simulink model "stewart_kinematics"  (R2018a)
settings: Solver=VariableStepAuto  StartTime=0.0  StopTime=1  FixedStep=1e-6  RelTol=1e-3  EnableMultiTasking=on
values from neighbouring files (symbols this model uses):
  stewart = initializeParameters(stewart)    [params_micro_hexapod.m]    (also in params_nano_hexapod.m; stewart_parameters.m = struct())
  X = dmax.*cos(repmat(phi,length(theta),1)).*cos(repmat(theta,length(phi),1))'    [Position_max.m]    (also in getMaxPositions.m)
  Y = dmax.*cos(repmat(phi,length(theta),1)).*sin(repmat(theta,length(phi),1))'    [Position_max.m]    (also in getMaxPositions.m)
  Z = dmax.*sin(repmat(phi,length(theta),1))    [Position_max.m]    (also in getMaxPositions.m)
undefined symbols (not defined in the file or in its folder): sample
libraries: sm_lib x118, nesl_utility x66, simulink x1
(part 1 of 5)
settings Model: Creator=ThomasDehaeze  LastModifiedBy=DEHAEZE
settings DataIOCC: SaveOutput=off  SignalLogging=off  DSMLogging=off  SaveTime=off
settings OptimizationCC: LifeSpan=inf
settings DebuggingCC: AllowSymbolicDim=off  SFUnexpectedBacktrackingDiag=warning  SFNoUnconditionalDefaultTransitionDiag=warning  SFExecutionAtInitializationDiag=none
settings CodeAppCC: StateflowObjectComments=on
settings GRTTargetCC: TargetLangStandard=C89/C90 (ANSI)  GeneratePreprocessorConditionals=Disable all
settings ConfigComp: CovMetricSettings=dw  CovHtmlReporting=on  CovSaveCumulativeToWorkspaceVar=on  CovSaveSingleToWorkspaceVar=on  CovExternalEMLEnable=off  CovSFcnEnable=off
settings SimscapeCC: SimscapeNominalValues="[{\"value\":\"10\",\"unit\":\"V\"},{\"value\":\"1\",\"unit\":\"A\"},{\"value\":\"10\",\"unit\":\"N*m\"},{\"value\":\"10\",\"unit\":\"bar\"},{\"value\":\"100\",\"unit\":\"kJ/kg\"},{\"value\":\"1\",\"unit\":\"kW\"},{\"value\":\"300\",\"unit\":\"K\"},{\"value\":\"100\",\"unit\":\"cm^3/s\"},{\"value\":\"1\",\"unit\":\"kN\"},{\"value\":\"1\",\"unit\":\"g/cm^3\"},{\"value\":\"1\",\"unit\":\"l\"},{\"value\":\"1\",\"unit\":\"cm^2\"},{\"value\":\"60\",\"unit\":\"Hz\"}]"  SimscapeLogType=all  SimscapeLogDataHistory=10000
settings ConfigurationSet: Description=SimMechanics 2G

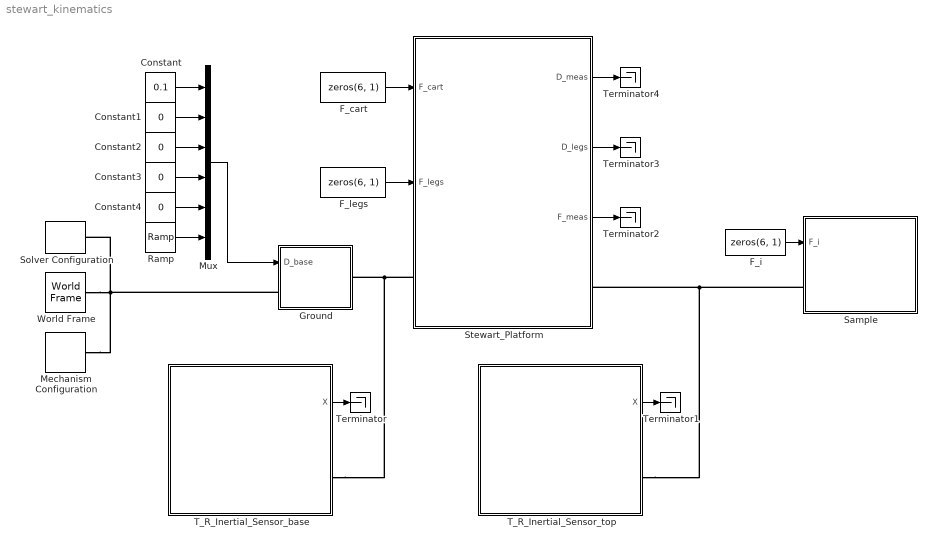
== system stewart_kinematics ==
  Constant : Constant  Value=0.1
  Constant{1..4} (4 alike) : Constant  Value=0
  F_cart : Constant  Value=zeros(6, 1)
  F_i : Constant  Value=zeros(6, 1)
  F_legs : Constant  Value=zeros(6, 1)
  Ground : Subsystem
  Mechanism Configuration : sm_lib/Utilities/Mechanism Configuration  UniformGravity=Constant  GravityVector=[0 0 0]  GravityUnits=m/s^2  LinearizationDelta=0.001
  Mux : Mux  Inputs=6
  Ramp : simulink/Sources/Ramp  slope=2*pi  start=0  InitialOutput=0
  Sample : Subsystem
      mask init:
      | load('./mat/sample.mat', 'sample');
  Solver Configuration : nesl_utility/Solver Configuration  PhysicalDomain=network_engine_domain  SubClassName=solver  LeftPortType=input  RightPortType=generic  Tones=[]  Harmonics=[]  SimulateNoise=off  Profile=off  UseLocalSampling=off  EnableSwitchedLinearOptims=on  FrequencyDomain=off  UseCCode=off  RelTol=0.001  AbsTol=1e-06  MinStep=1e-09  ToWorkspace=off  RevertToSquareIcSolve=off  NumHomotopyIterations=100  PhasorMode=off  PhasorModeNumHarmonics=1  DoDC=off  ResidualTolerance=1e-09  UseLocalSolver=off  LocalSolverChoice=NE_BACKWARD_EULER_ADVANCER  LocalSolverSampleTime=0.001  DoFixedCost=off  MaxNonlinIter=3  MaxModeIter=2  LinearAlgebra=Sparse  EquationFormulation=NE_TIME_EF  DelaysMemoryBudget=1024  AutomaticFiltering=on  FilteringTimeConstant=0.001
  Stewart_Platform : Subsystem
      mask init:
      | load('./mat/stewart.mat', 'stewart');
  T_R_Inertial_Sensor_base : Subsystem
  T_R_Inertial_Sensor_top : Subsystem
  Terminator{,1..4} (5 alike) : Terminator
  World Frame : sm_lib/Frames and Transforms/World Frame
  wires:
  F_cart/1 -> Stewart_Platform/1(F_cart)
  Stewart_Platform/1(D_meas) -> Terminator4/1
  Stewart_Platform/3(F_meas) -> Terminator2/1
  F_legs/1 -> Stewart_Platform/2(F_legs)
  Mux/1 -> Ground/1(D_base)
  F_i/1 -> Sample/1(F_i)
  T_R_Inertial_Sensor_base/1(X) -> Terminator/1
  T_R_Inertial_Sensor_top/1(X) -> Terminator1/1
  Stewart_Platform/2(D_legs) -> Terminator3/1
  Constant/1 -> Mux/1
  Constant1/1 -> Mux/2
  Constant2/1 -> Mux/3
  Constant3/1 -> Mux/4
  Constant4/1 -> Mux/5
  Ramp/1 -> Mux/6
  connections:
  Sample/LConn1 -- T_R_Inertial_Sensor_top/RConn1 -- Stewart_Platform/RConn1
  Mechanism Configuration/RConn1 -- Solver Configuration/RConn1 -- Ground/LConn1 -- World Frame/RConn1
  Stewart_Platform/LConn1 -- T_R_Inertial_Sensor_base/RConn1 -- Ground/RConn1

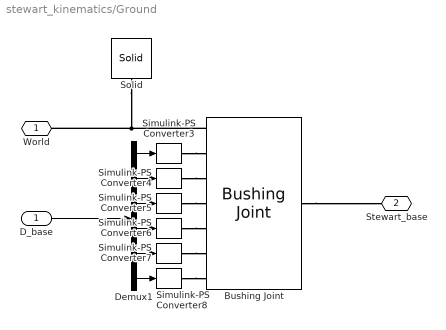
== system stewart_kinematics/Ground ==
  D_base : Inport
  Bushing Joint : sm_lib/Joints/Bushing Joint  SenseConstraintForce=off  SenseConstraintForceX=off  SenseConstraintForceY=off  SenseConstraintForceZ=off  SenseConstraintTorque=off  SenseConstraintTorqueX=off  SenseConstraintTorqueY=off  SenseConstraintTorqueZ=off  SenseTotalForce=off  SenseTotalForceX=off  SenseTotalForceY=off  SenseTotalForceZ=off  SenseTotalTorque=off  SenseTotalTorqueX=off  SenseTotalTorqueY=off  SenseTotalTorqueZ=off  CompositeWrenchDir=FollowerOnBase  CompositeWrenchFrame=BaseFrame  PxEquilibriumPosition=0  PxEquilibriumPositionUnits=m  PxSpringStiffness=0  PxSpringStiffnessUnits=N/m  PxDampingCoefficient=0  PxDampingCoefficientUnits=N/(m/s)  PxTorqueActuationMode=ComputedTorque  PxMotionActuationMode=InputMotion  PxSensePosition=off  PxSenseVelocity=off  PxSenseAcceleration=off  PxSenseTorqueForce=off  PxPositionTargetSpecify=off  PxPositionTargetPriority=High  PxPositionTargetValue=0  PxPositionTargetValueUnits=m  PxVelocityTargetSpecify=off  PxVelocityTargetPriority=High  PxVelocityTargetValue=0  PxVelocityTargetValueUnits=m/s  PyEquilibriumPosition=0  PyEquilibriumPositionUnits=m  PySpringStiffness=0  PySpringStiffnessUnits=N/m  PyDampingCoefficient=0  PyDampingCoefficientUnits=N/(m/s)  PyTorqueActuationMode=ComputedTorque  PyMotionActuationMode=InputMotion  PySensePosition=off  PySenseVelocity=off  PySenseAcceleration=off  PySenseTorqueForce=off  PyPositionTargetSpecify=off  PyPositionTargetPriority=High  PyPositionTargetValue=0  PyPositionTargetValueUnits=m  PyVelocityTargetSpecify=off  PyVelocityTargetPriority=High  PyVelocityTargetValue=0  PyVelocityTargetValueUnits=m/s  PzEquilibriumPosition=0  PzEquilibriumPositionUnits=m  PzSpringStiffness=0  PzSpringStiffnessUnits=N/m  PzDampingCoefficient=0  PzDampingCoefficientUnits=N/(m/s)  PzTorqueActuationMode=ComputedTorque  PzMotionActuationMode=InputMotion  PzSensePosition=off  PzSenseVelocity=off  PzSenseAcceleration=off  PzSenseTorqueForce=off  PzPositionTargetSpecify=off  PzPositionTargetPriority=High  PzPositionTargetValue=0  PzPositionTargetValueUnits=m  PzVelocityTargetSpecify=off  PzVelocityTargetPriority=High  PzVelocityTargetValue=0  PzVelocityTargetValueUnits=m/s  RxEquilibriumPosition=0  RxEquilibriumPositionUnits=deg  RxSpringStiffness=0  RxSpringStiffnessUnits=N*m/deg  RxDampingCoefficient=0  RxDampingCoefficientUnits=N*m/(deg/s)  RxTorqueActuationMode=ComputedTorque  RxMotionActuationMode=InputMotion  RxSensePosition=off  RxSenseVelocity=off  RxSenseAcceleration=off  RxSenseTorqueForce=off  RxPositionTargetSpecify=off  RxPositionTargetPriority=High  RxPositionTargetValue=0  RxPositionTargetValueUnits=deg  RxVelocityTargetSpecify=off  RxVelocityTargetPriority=High  RxVelocityTargetValue=0  RxVelocityTargetValueUnits=deg/s  RyEquilibriumPosition=0  RyEquilibriumPositionUnits=deg  RySpringStiffness=0  RySpringStiffnessUnits=N*m/deg  RyDampingCoefficient=0  RyDampingCoefficientUnits=N*m/(deg/s)  RyTorqueActuationMode=ComputedTorque  RyMotionActuationMode=InputMotion  RySensePosition=off  RySenseVelocity=off  RySenseAcceleration=off  RySenseTorqueForce=off  RyPositionTargetSpecify=off  RyPositionTargetPriority=High  RyPositionTargetValue=0  RyPositionTargetValueUnits=deg  RyVelocityTargetSpecify=off  RyVelocityTargetPriority=High  RyVelocityTargetValue=0  RyVelocityTargetValueUnits=deg/s  RzEquilibriumPosition=0  RzEquilibriumPositionUnits=deg  RzSpringStiffness=0  RzSpringStiffnessUnits=N*m/deg  RzDampingCoefficient=0  RzDampingCoefficientUnits=N*m/(deg/s)  RzTorqueActuationMode=ComputedTorque  RzMotionActuationMode=InputMotion  RzSensePosition=off  RzSenseVelocity=off  RzSenseAcceleration=off  RzSenseTorqueForce=off  RzPositionTargetSpecify=off  RzPositionTargetPriority=High  RzPositionTargetValue=0  RzPositionTargetValueUnits=deg  RzVelocityTargetSpecify=off  RzVelocityTargetPriority=High  RzVelocityTargetValue=0  RzVelocityTargetValueUnits=deg/s
      settings: SourceProductName=Simscape Multibody
  Demux1 : Demux  Outputs=6
  Simulink-PS Converter{3..8} (6 alike) : nesl_utility/Simulink-PS Converter  PhysicalDomain=network_engine_domain  SubClassName=ps_input  LeftPortType=input  RightPortType=output  PseudoPeriodic=off  Frequencies=[]  NoiseDistribution=none  NoiseParameters=[]  Unit=1  AffineConversion=off  FilteringAndDerivatives=filter  SimscapeFilterOrder=2  InputFilterTimeConstant=0.0001  UdotUserProvided=0
  Solid : sm_lib/Body Elements/Solid  InertiaType=CalculateFromGeometry  Mass=1  MassUnits=kg  CenterOfMass=[0 0 0]  CenterOfMassUnits=m  MomentsOfInertia=[1 1 1]  MomentsOfInertiaUnits=kg*m^2  ProductsOfInertia=[0 0 0]  ProductsOfInertiaUnits=kg*m^2  DensityBased=on  Density=1000  DensityUnits=kg/m^3  DoExposeReferenceFrame=off  SerializedFrames=<Frames><Frame><Id>Frame1</Id><Value><Name>F1</Name><Origin><Source>GeometricFeature</Source><FeatureName>top surface</FeatureName></Origin><PrimaryAxis><DefinedDirection>+Z</DefinedDirection><Source>ReferenceFrame</Source><SourceDirection>+Z</SourceDirection><FeatureName></FeatureName></PrimaryAxis><SecondaryAxis><DefinedDirection>+X</DefinedDirection><Source>ReferenceFrame</Source><SourceDirection>+X</SourceDirection><FeatureName></FeatureName></SecondaryAxis></Value></Frame></Frames>  GraphicType=FromGeometry  MarkerShape=Sphere  MarkerSize=10  GraphicVisPropType=SimpleVisualProperties  GraphicDiffuseColor=[0.5 0.5 0.5]  GraphicSpecularColor=[0.5 0.5 0.5 1.0]  GraphicAmbientColor=[0.15 0.15 0.15 1.0]  GraphicEmissiveColor=[0.0 0.0 0.0 1.0]  GraphicShininess=75  GraphicOpacity=1.0  GeometryShape=Cylinder  RectangleSize=[1 1]  RectangleSizeUnits=m  BrickDimensions=[1 1 0.1]  BrickDimensionUnits=m  CylinderRadius=0.5  CylinderRadiusUnits=m  CylinderLength=0.1  CylinderLengthUnits=m  SphereRadius=1  SphereRadiusUnits=m  EllipsoidRadii=[1 1 1]  EllipsoidRadiiUnits=m  ExtrusionCrossSection=[1 1; -1 1; -1 -1; 1 -1]  ExtrusionCrossSectionUnits=m  ExtrusionLength=1  ExtrusionLengthUnits=m  PolygonNumSides=3  PolygonOuterRadius=1  PolygonOuterRadiusUnits=m  ExtGeomFileType=STEP  ExtGeomFileUnits=m  RevolutionCrossSection=[1 1; 1 -1; 2 -1; 2 1]  RevolutionCrossSectionUnits=m  RevolutionExtent=Full  RevolutionAngle=180  RevolutionAngleUnits=deg
  World : PMIOPort  Side=Left
  Stewart_base : PMIOPort  Port=2  Side=Right
  wires:
  Demux1/1 -> Simulink-PS Converter3/1
  Demux1/2 -> Simulink-PS Converter4/1
  Demux1/3 -> Simulink-PS Converter5/1
  Demux1/4 -> Simulink-PS Converter6/1
  Demux1/5 -> Simulink-PS Converter7/1
  Demux1/6 -> Simulink-PS Converter8/1
  D_base/1 -> Demux1/1
  connections:
  Bushing Joint/RConn1 -- Stewart_base/RConn1
  Solid/LConn1 -- World/RConn1 -- Bushing Joint/LConn1
  Simulink-PS Converter3/RConn1 -- Bushing Joint/LConn2
  Simulink-PS Converter4/RConn1 -- Bushing Joint/LConn3
  Simulink-PS Converter5/RConn1 -- Bushing Joint/LConn4
  Simulink-PS Converter8/RConn1 -- Bushing Joint/LConn7
  Simulink-PS Converter7/RConn1 -- Bushing Joint/LConn6
  Simulink-PS Converter6/RConn1 -- Bushing Joint/LConn5

== system stewart_kinematics/Sample ==
  note: Sample
  note: X-Offset for the Sample
  F_i : Inport
  Eternal_Force_and_Torque : Subsystem
  Rigid Transform : sm_lib/Frames and Transforms/Rigid Transform  TranslationMethod=StandardAxis  TranslationStandardOffset=sample.offset  TranslationLengthUnit=mm  TranslationStandardAxis=+X  TranslationCartesianOffset=[0 0 0]  TranslationROffset=0  TranslationROffsetUnits=m  TranslationZOffset=0  TranslationZOffsetUnits=m  TranslationThetaOffset=0  TranslationThetaOffsetUnits=deg  RotationMethod=None  RotationAngleUnits=deg  RotationStandardAxis=+Z  RotationAngle=0.0  RotationArbitraryAxis=[0 0 1]  FollAlignAxisA=+X  BaseAlignAxisA=+Y  FollAlignAxisB=+Y  BaseAlignAxisB=+Z  RotationSequenceAxes=FollowerAxes  RotationSequence=XYX  RotationSequenceAngles=[0 0 0]  RotationSequenceAnglesUnits=deg  RotationMatrix=[1 0 0; 0 1 0; 0 0 1]
  Solid1 : sm_lib/Body Elements/Solid  InertiaType=CalculateFromGeometry  Mass=sample.mass  MassUnits=kg  CenterOfMass=[0 0 0]  CenterOfMassUnits=m  MomentsOfInertia=[1 1 1]  MomentsOfInertiaUnits=kg*m^2  ProductsOfInertia=[1 1 1]  ProductsOfInertiaUnits=kg*m^2  DensityBased=off  Density=1000  DensityUnits=kg/m^3  DoExposeReferenceFrame=on  SerializedFrames=<Frames><Frame><Id>Frame1</Id><Value><Name>F1</Name><Origin><Source>GeometricFeature</Source><FeatureName>bottom surface</FeatureName></Origin><PrimaryAxis><DefinedDirection>+Z</DefinedDirection><Source>ReferenceFrame</Source><SourceDirection>+Z</SourceDirection><FeatureName></FeatureName></PrimaryAxis><SecondaryAxis><DefinedDirection>+X</DefinedDirection><Source>ReferenceFrame</Source><SourceDirection>+X</SourceDirection><FeatureName></FeatureName></SecondaryAxis></Value></Frame></Frames>  GraphicType=FromGeometry  MarkerShape=Sphere  MarkerSize=10  GraphicVisPropType=SimpleVisualProperties  GraphicDiffuseColor=sample.color  GraphicSpecularColor=[0.5 0.5 0.5 1.0]  GraphicAmbientColor=[0.15 0.15 0.15 1.0]  GraphicEmissiveColor=[0.0 0.0 0.0 1.0]  GraphicShininess=75  GraphicOpacity=1.0  GeometryShape=Cylinder  RectangleSize=[1 1]  RectangleSizeUnits=m  BrickDimensions=[1 1 1]  BrickDimensionUnits=m  CylinderRadius=sample.radius  CylinderRadiusUnits=mm  CylinderLength=sample.height  CylinderLengthUnits=mm  SphereRadius=1  SphereRadiusUnits=m  EllipsoidRadii=[1 1 1]  EllipsoidRadiiUnits=m  ExtrusionCrossSection=[1 1; -1 1; -1 -1; 1 -1]  ExtrusionCrossSectionUnits=m  ExtrusionLength=1  ExtrusionLengthUnits=m  PolygonNumSides=3  PolygonOuterRadius=1  PolygonOuterRadiusUnits=m  ExtGeomFileType=STEP  ExtGeomFileUnits=m  RevolutionCrossSection=[1 1; 1 -1; 2 -1; 2 1]  RevolutionCrossSectionUnits=m  RevolutionExtent=Full  RevolutionAngle=180  RevolutionAngleUnits=deg
  Sample_bot : PMIOPort  Side=Left
  wires:
  F_i/1 -> Eternal_Force_and_Torque/1(F_ext)
  connections:
  Solid1/LConn1 -- Rigid Transform/RConn1
  Sample_bot/RConn1 -- Rigid Transform/LConn1
  Eternal_Force_and_Torque/RConn1 -- Solid1/RConn1

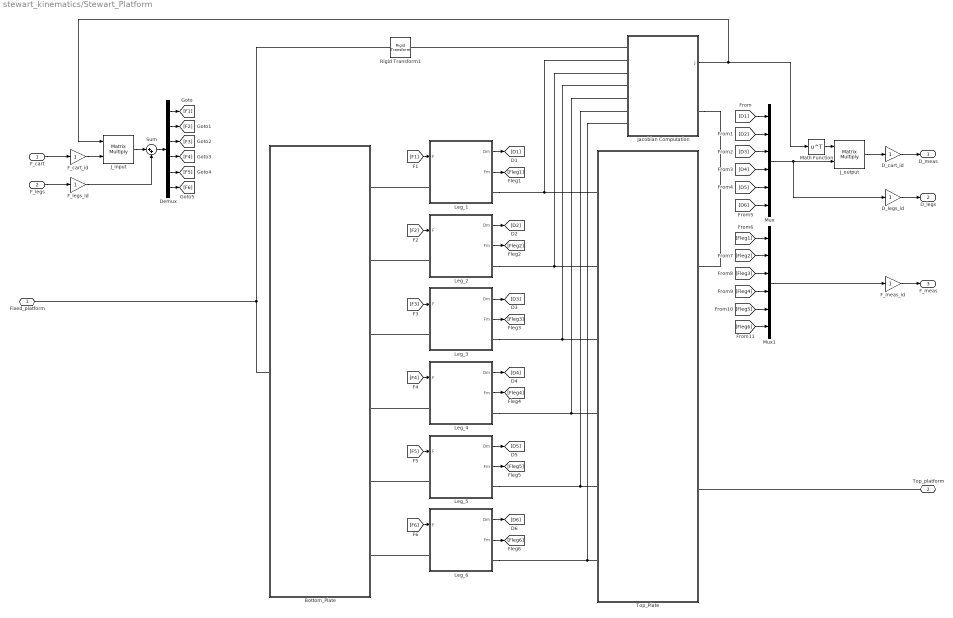
== system stewart_kinematics/Stewart_Platform ==
  F_cart : Inport
  F_legs : Inport  Port=2
  Bottom_Plate : Subsystem
  D_cart_id : Gain
  D_legs_id : Gain
  Demux : Demux  Outputs=6
  F_cart_id : Gain
  F_legs_id : Gain
  F_meas_id : Gain
  J_input : Product  Multiplication=Matrix(*)
  J_output : Product  Multiplication=Matrix(*)
  Jacobian Computation : Subsystem
  Leg_1 : Subsystem
  Leg_2 : Subsystem
  Leg_3 : Subsystem
  Leg_4 : Subsystem
  Leg_5 : Subsystem
  Leg_6 : Subsystem
  Math Function : Math  Operator=transpose  SaturateOnIntegerOverflow=on
  Mux : Mux  Inputs=6
  Mux1 : Mux  Inputs=6
  Rigid Transform1 : sm_lib/Frames and Transforms/Rigid Transform  TranslationMethod=StandardAxis  TranslationStandardOffset=stewart.jacobian+stewart.h  TranslationLengthUnit=mm  TranslationStandardAxis=+Z  TranslationCartesianOffset=[0 0 0]  TranslationROffset=0  TranslationROffsetUnits=m  TranslationZOffset=0  TranslationZOffsetUnits=m  TranslationThetaOffset=0  TranslationThetaOffsetUnits=deg  RotationMethod=None  RotationAngleUnits=deg  RotationStandardAxis=+Z  RotationAngle=0.0  RotationArbitraryAxis=[0 0 1]  FollAlignAxisA=+X  BaseAlignAxisA=+Y  FollAlignAxisB=+Y  BaseAlignAxisB=+Z  RotationSequenceAxes=FollowerAxes  RotationSequence=XYX  RotationSequenceAngles=[0 0 0]  RotationSequenceAnglesUnits=deg  RotationMatrix=[1 0 0; 0 1 0; 0 0 1]
  Sum : Sum  Inputs=|++
  Top_Plate : Subsystem
  Fixed_platform : PMIOPort  Side=Left
  Top_platform : PMIOPort  Port=2  Side=Right
  D_meas : Outport
  D_legs : Outport  Port=2
  F_meas : Outport  Port=3
  wires:
  Demux/1 -> [F1]
  [F3] -> Leg_3/1(F)
  [F5] -> Leg_5/1(F)
  Demux/4 -> [F4]
  Demux/2 -> [F2]
  Leg_5/1(Dm) -> [D5]
  Leg_3/1(Dm) -> [D3]
  Demux/5 -> [F5]
  Demux/6 -> [F6]
  [F6] -> Leg_6/1(F)
  [F4] -> Leg_4/1(F)
  Demux/3 -> [F3]
  Leg_4/1(Dm) -> [D4]
  Leg_2/1(Dm) -> [D2]
  [F2] -> Leg_2/1(F)
  Leg_6/1(Dm) -> [D6]
  F_cart/1 -> F_cart_id/1
  Jacobian Computation/1(J) -> J_input/1, Math Function/1
  J_input/1 -> Sum/1
  [D3] -> Mux/3
  J_output/1 -> D_cart_id/1
  [D5] -> Mux/5
  Mux/1 -> D_legs_id/1, J_output/2
  Math Function/1 -> J_output/1
  [D6] -> Mux/6
  [D1] -> Mux/1
  [D4] -> Mux/4
  [D2] -> Mux/2
  [F1] -> Leg_1/1(F)
  Leg_1/1(Dm) -> [D1]
  Sum/1 -> Demux/1
  F_legs/1 -> F_legs_id/1
  D_legs_id/1 -> D_legs/1
  D_cart_id/1 -> D_meas/1
  F_legs_id/1 -> Sum/2
  F_cart_id/1 -> J_input/2
  Leg_2/2(Fm) -> [Fleg2]
  Leg_3/2(Fm) -> [Fleg3]
  Leg_4/2(Fm) -> [Fleg4]
  Leg_5/2(Fm) -> [Fleg5]
  Leg_6/2(Fm) -> [Fleg6]
  Leg_1/2(Fm) -> [Fleg1]
  [Fleg1] -> Mux1/1
  [Fleg2] -> Mux1/2
  [Fleg3] -> Mux1/3
  [Fleg4] -> Mux1/4
  [Fleg5] -> Mux1/5
  [Fleg6] -> Mux1/6
  F_meas_id/1 -> F_meas/1
  Mux1/1 -> F_meas_id/1
  connections:
  Jacobian Computation/LConn3 -- Leg_2/RConn1 -- Top_Plate/LConn2
  Leg_4/LConn1 -- Bottom_Plate/RConn4
  Jacobian Computation/LConn5 -- Leg_4/RConn1 -- Top_Plate/LConn4
  Top_Plate/LConn1 -- Leg_1/RConn1 -- Jacobian Computation/LConn2
  Leg_3/LConn1 -- Bottom_Plate/RConn3
  Jacobian Computation/LConn4 -- Top_Plate/LConn3 -- Leg_3/RConn1
  Jacobian Computation/LConn6 -- Leg_5/RConn1 -- Top_Plate/LConn5
  Leg_2/LConn1 -- Bottom_Plate/RConn2
  Leg_5/LConn1 -- Bottom_Plate/RConn5
  Leg_1/LConn1 -- Bottom_Plate/RConn1
  Jacobian Computation/LConn7 -- Leg_6/RConn1 -- Top_Plate/LConn6
  Leg_6/LConn1 -- Bottom_Plate/RConn6
  Top_platform/RConn1 -- Top_Plate/RConn2
  Jacobian Computation/RConn1 -- Top_Plate/RConn1
  Rigid Transform1/LConn1 -- Bottom_Plate/LConn1 -- Fixed_platform/RConn1
  Jacobian Computation/LConn1 -- Rigid Transform1/RConn1

== system stewart_kinematics/T_R_Inertial_Sensor_base ==
  Model : ModelReference  ModelNameDialog=QuaternionToAngles.slx  SimulationMode=Normal  ModelReferenceVersion=1.10
  Mux : Mux  Inputs=6
  PS-Simulink Converter{1,3..5} (4 alike) : nesl_utility/PS-Simulink Converter  PhysicalDomain=network_engine_domain  SubClassName=ps_output  LeftPortType=input  RightPortType=output  PseudoPeriodic=off  Frequencies=[]  Unit=1  AffineConversion=off
  Transform Sensor : sm_lib/Frames and Transforms/Transform Sensor  MeasurementFrame=Base  SenseAngle=off  SenseAxis=off  SenseAngle1=off  SenseAngle2=off  SenseAngle3=off  SenseQ=on  SenseR=off  SenseOmegaX=off  SenseOmegaY=off  SenseOmegaZ=off  SenseOmega1=off  SenseOmega2=off  SenseOmega3=off  SenseQDot=off  SenseRDot=off  SenseAlphaX=off  SenseAlphaY=off  SenseAlphaZ=off  SenseAlpha1=off  SenseAlpha2=off  SenseAlpha3=off  SenseQDDot=off  SenseRDDot=off  SenseX=on  SenseY=on  SenseZ=on  SenseRad=off  SenseAzim=off  SenseDist=off  SenseInc=off  SenseXDot=off  SenseYDot=off  SenseZDot=off  SenseRadDot=off  SenseAzimDot=off  SenseDistDot=off  SenseIncDot=off  SenseXDDot=off  SenseYDDot=off  SenseZDDot=off  SenseRadDDot=off  SenseAzimDDot=off  SenseDistDDot=off  SenseIncDDot=off
  World Frame1 : sm_lib/Frames and Transforms/World Frame
  F : PMIOPort  Side=Right
  X : Outport
  wires:
  PS-Simulink Converter4/1 -> Mux/2  "y"
  PS-Simulink Converter3/1 -> Mux/1  "x"
  PS-Simulink Converter1/1 -> Model/1
  Model/1 -> Mux/4
  Model/2 -> Mux/5
  Model/3 -> Mux/6
  PS-Simulink Converter5/1 -> Mux/3  "z"
  Mux/1 -> X/1
  connections:
  World Frame1/RConn1 -- Transform Sensor/LConn1
  Transform Sensor/RConn1 -- F/RConn1
  Transform Sensor/RConn5 -- PS-Simulink Converter5/LConn1
  Transform Sensor/RConn3 -- PS-Simulink Converter3/LConn1
  Transform Sensor/RConn4 -- PS-Simulink Converter4/LConn1
  PS-Simulink Converter1/LConn1 -- Transform Sensor/RConn2

== system stewart_kinematics/T_R_Inertial_Sensor_top ==
  Model : ModelReference  ModelNameDialog=QuaternionToAngles.slx  SimulationMode=Normal  ModelReferenceVersion=1.10
  Mux : Mux  Inputs=6
  PS-Simulink Converter{1,3..5} (4 alike) : nesl_utility/PS-Simulink Converter  PhysicalDomain=network_engine_domain  SubClassName=ps_output  LeftPortType=input  RightPortType=output  PseudoPeriodic=off  Frequencies=[]  Unit=1  AffineConversion=off
  Transform Sensor : sm_lib/Frames and Transforms/Transform Sensor  MeasurementFrame=Base  SenseAngle=off  SenseAxis=off  SenseAngle1=off  SenseAngle2=off  SenseAngle3=off  SenseQ=on  SenseR=off  SenseOmegaX=off  SenseOmegaY=off  SenseOmegaZ=off  SenseOmega1=off  SenseOmega2=off  SenseOmega3=off  SenseQDot=off  SenseRDot=off  SenseAlphaX=off  SenseAlphaY=off  SenseAlphaZ=off  SenseAlpha1=off  SenseAlpha2=off  SenseAlpha3=off  SenseQDDot=off  SenseRDDot=off  SenseX=on  SenseY=on  SenseZ=on  SenseRad=off  SenseAzim=off  SenseDist=off  SenseInc=off  SenseXDot=off  SenseYDot=off  SenseZDot=off  SenseRadDot=off  SenseAzimDot=off  SenseDistDot=off  SenseIncDot=off  SenseXDDot=off  SenseYDDot=off  SenseZDDot=off  SenseRadDDot=off  SenseAzimDDot=off  SenseDistDDot=off  SenseIncDDot=off
  World Frame1 : sm_lib/Frames and Transforms/World Frame
  F : PMIOPort  Side=Right
  X : Outport
  wires:
  Mux/1 -> X/1
  PS-Simulink Converter5/1 -> Mux/3  "z"
  Model/3 -> Mux/6
  Model/2 -> Mux/5
  Model/1 -> Mux/4
  PS-Simulink Converter1/1 -> Model/1
  PS-Simulink Converter3/1 -> Mux/1  "x"
  PS-Simulink Converter4/1 -> Mux/2  "y"
  connections:
  PS-Simulink Converter1/LConn1 -- Transform Sensor/RConn2
  Transform Sensor/RConn4 -- PS-Simulink Converter4/LConn1
  Transform Sensor/RConn3 -- PS-Simulink Converter3/LConn1
  Transform Sensor/RConn5 -- PS-Simulink Converter5/LConn1
  Transform Sensor/RConn1 -- F/RConn1
  World Frame1/RConn1 -- Transform Sensor/LConn1

== system stewart_kinematics/Sample/Eternal_Force_and_Torque ==
  F_ext : Inport  PortDimensions=6
  Demux1 : Demux  Outputs=6
  External Force and Torque1 : sm_lib/Forces and Torques/External Force and Torque  ForceResolutionFrame=World  EnableForceX=on  EnableForceY=on  EnableForceZ=on  EnableForce=off  TorqueResolutionFrame=AttachedFrame  EnableTorqueX=on  EnableTorqueY=on  EnableTorqueZ=on  EnableTorque=off
  Simulink-PS Converter{1..6} (6 alike) : nesl_utility/Simulink-PS Converter  PhysicalDomain=network_engine_domain  SubClassName=ps_input  LeftPortType=input  RightPortType=output  PseudoPeriodic=off  Frequencies=[]  NoiseDistribution=none  NoiseParameters=[]  Unit=1  AffineConversion=off  FilteringAndDerivatives=provide  SimscapeFilterOrder=1  InputFilterTimeConstant=0.001  UdotUserProvided=0
  F : PMIOPort  Side=Right
  wires:
  Demux1/2 -> Simulink-PS Converter4/1
  Demux1/1 -> Simulink-PS Converter3/1
  Demux1/3 -> Simulink-PS Converter5/1
  F_ext/1 -> Demux1/1
  Demux1/6 -> Simulink-PS Converter6/1
  Demux1/4 -> Simulink-PS Converter1/1
  Demux1/5 -> Simulink-PS Converter2/1
  connections:
  F/RConn1 -- External Force and Torque1/RConn1
  Simulink-PS Converter4/RConn1 -- External Force and Torque1/LConn2
  Simulink-PS Converter5/RConn1 -- External Force and Torque1/LConn3
  Simulink-PS Converter3/RConn1 -- External Force and Torque1/LConn1
  Simulink-PS Converter1/RConn1 -- External Force and Torque1/LConn4
  Simulink-PS Converter2/RConn1 -- External Force and Torque1/LConn5
  Simulink-PS Converter6/RConn1 -- External Force and Torque1/LConn6

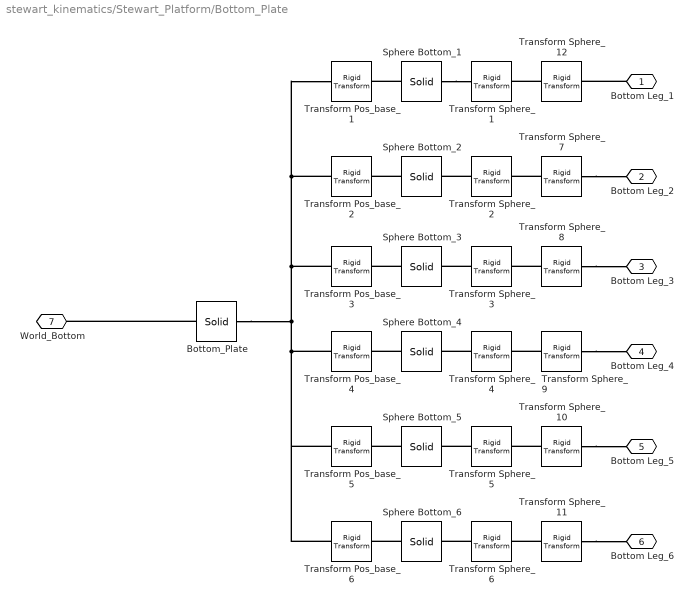
== system stewart_kinematics/Stewart_Platform/Bottom_Plate ==
  Bottom_Plate : sm_lib/Body Elements/Solid  InertiaType=CalculateFromGeometry  Mass=1  MassUnits=kg  CenterOfMass=[0 0 0]  CenterOfMassUnits=m  MomentsOfInertia=[1 1 1]  MomentsOfInertiaUnits=kg*m^2  ProductsOfInertia=[1 1 1]  ProductsOfInertiaUnits=kg*m^2  DensityBased=on  Density=stewart.BP.density  DensityUnits=kg/m^3  DoExposeReferenceFrame=on  SerializedFrames=<Frames><Frame><Id>Frame1</Id><Value><Name>T</Name><Origin><Source>GeometricFeature</Source><FeatureName>side surface 4</FeatureName></Origin><PrimaryAxis><DefinedDirection>+Z</DefinedDirection><Source>ReferenceFrame</Source><SourceDirection>+Z</SourceDirection><FeatureName></FeatureName></PrimaryAxis><SecondaryAxis><DefinedDirection>+X</DefinedDirection><Source>ReferenceFrame</Source><SourceDirection>+X</SourceDirection><FeatureName></FeatureName></SecondaryAxis></Value></Frame></Frames>  GraphicType=FromGeometry  MarkerShape=Sphere  MarkerSize=10  GraphicVisPropType=SimpleVisualProperties  GraphicDiffuseColor=stewart.BP.color  GraphicSpecularColor=[0.5 0.5 0.5 1.0]  GraphicAmbientColor=[0.15 0.15 0.15 1.0]  GraphicEmissiveColor=[0.0 0.0 0.0 1.0]  GraphicShininess=75  GraphicOpacity=1.0  GeometryShape=GeneralSolidOfRevolution  RectangleSize=[1 1]  RectangleSizeUnits=m  BrickDimensions=[1 1 1]  BrickDimensionUnits=m  CylinderRadius=1  CylinderRadiusUnits=m  CylinderLength=1  CylinderLengthUnits=m  SphereRadius=1  SphereRadiusUnits=m  EllipsoidRadii=[1 1 1]  EllipsoidRadiiUnits=m  ExtrusionCrossSection=[1 1; -1 1; -1 -1; 1 -1]  ExtrusionCrossSectionUnits=m  ExtrusionLength=1  ExtrusionLengthUnits=m  PolygonNumSides=3  PolygonOuterRadius=1  PolygonOuterRadiusUnits=m  ExtGeomFileType=STEP  ExtGeomFileUnits=m  RevolutionCrossSection=stewart.BP.shape  RevolutionCrossSectionUnits=mm  RevolutionExtent=Full  RevolutionAngle=180  RevolutionAngleUnits=deg
  Sphere Bottom_{1..6} (6 alike) : sm_lib/Body Elements/Solid  InertiaType=CalculateFromGeometry  Mass=1  MassUnits=kg  CenterOfMass=[0 0 0]  CenterOfMassUnits=m  MomentsOfInertia=[1 1 1]  MomentsOfInertiaUnits=kg*m^2  ProductsOfInertia=[1 1 1]  ProductsOfInertiaUnits=kg*m^2  DensityBased=on  Density=stewart.SP.density.bottom  DensityUnits=kg/m^3  DoExposeReferenceFrame=on  SerializedFrames=<Frames><Frame><Id>Frame1</Id><Value><Name>R1</Name><Origin><Source>ReferenceFrame</Source><FeatureName></FeatureName></Origin><PrimaryAxis><DefinedDirection>+Z</DefinedDirection><Source>ReferenceFrame</Source><SourceDirection>+Z</SourceDirection><FeatureName></FeatureName></PrimaryAxis><SecondaryAxis><DefinedDirection>+X</DefinedDirection><Source>ReferenceFrame</Source><SourceDirection>+X</SourceDirection><FeatureName></FeatureName></SecondaryAxis></Value></Frame></Frames>  GraphicType=FromGeometry  MarkerShape=Sphere  MarkerSize=10  GraphicVisPropType=SimpleVisualProperties  GraphicDiffuseColor=stewart.SP.color.bottom  GraphicSpecularColor=[0.5 0.5 0.5 1.0]  GraphicAmbientColor=[0.15 0.15 0.15 1.0]  GraphicEmissiveColor=[0.0 0.0 0.0 1.0]  GraphicShininess=75  GraphicOpacity=1.0  GeometryShape=GeneralSolidOfRevolution  RectangleSize=[1 1]  RectangleSizeUnits=m  BrickDimensions=[1 1 1]  BrickDimensionUnits=m  CylinderRadius=1  CylinderRadiusUnits=m  CylinderLength=1  CylinderLengthUnits=m  SphereRadius=1  SphereRadiusUnits=m  EllipsoidRadii=[1 1 1]  EllipsoidRadiiUnits=m  ExtrusionCrossSection=[1 1; -1 1; -1 -1; 1 -1]  ExtrusionCrossSectionUnits=m  ExtrusionLength=1  ExtrusionLengthUnits=m  PolygonNumSides=3  PolygonOuterRadius=1  PolygonOuterRadiusUnits=m  ExtGeomFileType=STEP  ExtGeomFileUnits=m  RevolutionCrossSection=stewart.Leg.support.bottom  RevolutionCrossSectionUnits=mm  RevolutionExtent=Full  RevolutionAngle=180  RevolutionAngleUnits=deg
  Transform Pos_base_1 : sm_lib/Frames and Transforms/Rigid Transform  TranslationMethod=Cartesian  TranslationStandardOffset=0  TranslationLengthUnit=m  TranslationStandardAxis=+Z  TranslationCartesianOffset=stewart.pos_base(1,:)  TranslationROffset=140  TranslationROffsetUnits=mm  TranslationZOffset=0  TranslationZOffsetUnits=m  TranslationThetaOffset=0  TranslationThetaOffsetUnits=deg  RotationMethod=None  RotationAngleUnits=deg  RotationStandardAxis=+Z  RotationAngle=0.0  RotationArbitraryAxis=[0 0 1]  FollAlignAxisA=+X  BaseAlignAxisA=+Y  FollAlignAxisB=+Y  BaseAlignAxisB=+Z  RotationSequenceAxes=FollowerAxes  RotationSequence=XYX  RotationSequenceAngles=[0 0 0]  RotationSequenceAnglesUnits=deg  RotationMatrix=[1 0 0; 0 1 0; 0 0 1]
  Transform Pos_base_2 : sm_lib/Frames and Transforms/Rigid Transform  TranslationMethod=Cartesian  TranslationStandardOffset=0  TranslationLengthUnit=m  TranslationStandardAxis=+Z  TranslationCartesianOffset=stewart.pos_base(2,:)  TranslationROffset=140  TranslationROffsetUnits=mm  TranslationZOffset=0  TranslationZOffsetUnits=m  TranslationThetaOffset=0  TranslationThetaOffsetUnits=deg  RotationMethod=None  RotationAngleUnits=deg  RotationStandardAxis=+Z  RotationAngle=0.0  RotationArbitraryAxis=[0 0 1]  FollAlignAxisA=+X  BaseAlignAxisA=+Y  FollAlignAxisB=+Y  BaseAlignAxisB=+Z  RotationSequenceAxes=FollowerAxes  RotationSequence=XYX  RotationSequenceAngles=[0 0 0]  RotationSequenceAnglesUnits=deg  RotationMatrix=[1 0 0; 0 1 0; 0 0 1]
  Transform Pos_base_3 : sm_lib/Frames and Transforms/Rigid Transform  TranslationMethod=Cartesian  TranslationStandardOffset=0  TranslationLengthUnit=m  TranslationStandardAxis=+Z  TranslationCartesianOffset=stewart.pos_base(3,:)  TranslationROffset=140  TranslationROffsetUnits=mm  TranslationZOffset=0  TranslationZOffsetUnits=m  TranslationThetaOffset=0  TranslationThetaOffsetUnits=deg  RotationMethod=None  RotationAngleUnits=deg  RotationStandardAxis=+Z  RotationAngle=0.0  RotationArbitraryAxis=[0 0 1]  FollAlignAxisA=+X  BaseAlignAxisA=+Y  FollAlignAxisB=+Y  BaseAlignAxisB=+Z  RotationSequenceAxes=FollowerAxes  RotationSequence=XYX  RotationSequenceAngles=[0 0 0]  RotationSequenceAnglesUnits=deg  RotationMatrix=[1 0 0; 0 1 0; 0 0 1]
  Transform Pos_base_4 : sm_lib/Frames and Transforms/Rigid Transform  TranslationMethod=Cartesian  TranslationStandardOffset=0  TranslationLengthUnit=m  TranslationStandardAxis=+Z  TranslationCartesianOffset=stewart.pos_base(4,:)  TranslationROffset=140  TranslationROffsetUnits=mm  TranslationZOffset=0  TranslationZOffsetUnits=m  TranslationThetaOffset=0  TranslationThetaOffsetUnits=deg  RotationMethod=None  RotationAngleUnits=deg  RotationStandardAxis=+Z  RotationAngle=0.0  RotationArbitraryAxis=[0 0 1]  FollAlignAxisA=+X  BaseAlignAxisA=+Y  FollAlignAxisB=+Y  BaseAlignAxisB=+Z  RotationSequenceAxes=FollowerAxes  RotationSequence=XYX  RotationSequenceAngles=[0 0 0]  RotationSequenceAnglesUnits=deg  RotationMatrix=[1 0 0; 0 1 0; 0 0 1]
  Transform Pos_base_5 : sm_lib/Frames and Transforms/Rigid Transform  TranslationMethod=Cartesian  TranslationStandardOffset=0  TranslationLengthUnit=m  TranslationStandardAxis=+Z  TranslationCartesianOffset=stewart.pos_base(5,:)  TranslationROffset=140  TranslationROffsetUnits=mm  TranslationZOffset=0  TranslationZOffsetUnits=m  TranslationThetaOffset=0  TranslationThetaOffsetUnits=deg  RotationMethod=None  RotationAngleUnits=deg  RotationStandardAxis=+Z  RotationAngle=0.0  RotationArbitraryAxis=[0 0 1]  FollAlignAxisA=+X  BaseAlignAxisA=+Y  FollAlignAxisB=+Y  BaseAlignAxisB=+Z  RotationSequenceAxes=FollowerAxes  RotationSequence=XYX  RotationSequenceAngles=[0 0 0]  RotationSequenceAnglesUnits=deg  RotationMatrix=[1 0 0; 0 1 0; 0 0 1]
  Transform Pos_base_6 : sm_lib/Frames and Transforms/Rigid Transform  TranslationMethod=Cartesian  TranslationStandardOffset=0  TranslationLengthUnit=m  TranslationStandardAxis=+Z  TranslationCartesianOffset=stewart.pos_base(6,:)  TranslationROffset=140  TranslationROffsetUnits=mm  TranslationZOffset=0  TranslationZOffsetUnits=m  TranslationThetaOffset=0  TranslationThetaOffsetUnits=deg  RotationMethod=None  RotationAngleUnits=deg  RotationStandardAxis=+Z  RotationAngle=0.0  RotationArbitraryAxis=[0 0 1]  FollAlignAxisA=+X  BaseAlignAxisA=+Y  FollAlignAxisB=+Y  BaseAlignAxisB=+Z  RotationSequenceAxes=FollowerAxes  RotationSequence=XYX  RotationSequenceAngles=[0 0 0]  RotationSequenceAnglesUnits=deg  RotationMatrix=[1 0 0; 0 1 0; 0 0 1]
  Transform Sphere_{1..6} (6 alike) : sm_lib/Frames and Transforms/Rigid Transform  TranslationMethod=Cartesian  TranslationStandardOffset=0  TranslationLengthUnit=mm  TranslationStandardAxis=+Z  TranslationCartesianOffset=[0 0 stewart.Leg.sphere.bottom+stewart.SP.thickness.bottom]  TranslationROffset=140  TranslationROffsetUnits=m  TranslationZOffset=0  TranslationZOffsetUnits=m  TranslationThetaOffset=0  TranslationThetaOffsetUnits=deg  RotationMethod=None  RotationAngleUnits=deg  RotationStandardAxis=+Z  RotationAngle=30  RotationArbitraryAxis=0  FollAlignAxisA=+X  BaseAlignAxisA=+Y  FollAlignAxisB=+Y  BaseAlignAxisB=+Z  RotationSequenceAxes=BaseAxes  RotationSequence=XYX  RotationSequenceAngles=[0 0 0]  RotationSequenceAnglesUnits=deg  RotationMatrix=0
  Transform Sphere_10 : sm_lib/Frames and Transforms/Rigid Transform  TranslationMethod=None  TranslationStandardOffset=0  TranslationLengthUnit=mm  TranslationStandardAxis=+Z  TranslationCartesianOffset=0  TranslationROffset=140  TranslationROffsetUnits=m  TranslationZOffset=0  TranslationZOffsetUnits=m  TranslationThetaOffset=0  TranslationThetaOffsetUnits=deg  RotationMethod=RotationMatrix  RotationAngleUnits=deg  RotationStandardAxis=+Z  RotationAngle=30  RotationArbitraryAxis=0  FollAlignAxisA=+X  BaseAlignAxisA=+Y  FollAlignAxisB=+Y  BaseAlignAxisB=+Z  RotationSequenceAxes=BaseAxes  RotationSequence=XYX  RotationSequenceAngles=[0 0 0]  RotationSequenceAnglesUnits=deg  RotationMatrix=stewart.lower_leg(5).rotation
  Transform Sphere_11 : sm_lib/Frames and Transforms/Rigid Transform  TranslationMethod=None  TranslationStandardOffset=0  TranslationLengthUnit=mm  TranslationStandardAxis=+Z  TranslationCartesianOffset=0  TranslationROffset=140  TranslationROffsetUnits=m  TranslationZOffset=0  TranslationZOffsetUnits=m  TranslationThetaOffset=0  TranslationThetaOffsetUnits=deg  RotationMethod=RotationMatrix  RotationAngleUnits=deg  RotationStandardAxis=+Z  RotationAngle=30  RotationArbitraryAxis=0  FollAlignAxisA=+X  BaseAlignAxisA=+Y  FollAlignAxisB=+Y  BaseAlignAxisB=+Z  RotationSequenceAxes=BaseAxes  RotationSequence=XYX  RotationSequenceAngles=[0 0 0]  RotationSequenceAnglesUnits=deg  RotationMatrix=stewart.lower_leg(6).rotation
  Transform Sphere_12 : sm_lib/Frames and Transforms/Rigid Transform  TranslationMethod=None  TranslationStandardOffset=0  TranslationLengthUnit=mm  TranslationStandardAxis=+Z  TranslationCartesianOffset=0  TranslationROffset=140  TranslationROffsetUnits=m  TranslationZOffset=0  TranslationZOffsetUnits=m  TranslationThetaOffset=0  TranslationThetaOffsetUnits=deg  RotationMethod=RotationMatrix  RotationAngleUnits=deg  RotationStandardAxis=+Z  RotationAngle=30  RotationArbitraryAxis=0  FollAlignAxisA=+X  BaseAlignAxisA=+Y  FollAlignAxisB=+Y  BaseAlignAxisB=+Z  RotationSequenceAxes=BaseAxes  RotationSequence=XYX  RotationSequenceAngles=[0 0 0]  RotationSequenceAnglesUnits=deg  RotationMatrix=stewart.lower_leg(1).rotation
  Transform Sphere_7 : sm_lib/Frames and Transforms/Rigid Transform  TranslationMethod=None  TranslationStandardOffset=0  TranslationLengthUnit=mm  TranslationStandardAxis=+Z  TranslationCartesianOffset=0  TranslationROffset=140  TranslationROffsetUnits=m  TranslationZOffset=0  TranslationZOffsetUnits=m  TranslationThetaOffset=0  TranslationThetaOffsetUnits=deg  RotationMethod=RotationMatrix  RotationAngleUnits=deg  RotationStandardAxis=+Z  RotationAngle=30  RotationArbitraryAxis=0  FollAlignAxisA=+X  BaseAlignAxisA=+Y  FollAlignAxisB=+Y  BaseAlignAxisB=+Z  RotationSequenceAxes=BaseAxes  RotationSequence=XYX  RotationSequenceAngles=[0 0 0]  RotationSequenceAnglesUnits=deg  RotationMatrix=stewart.lower_leg(2).rotation
  Transform Sphere_8 : sm_lib/Frames and Transforms/Rigid Transform  TranslationMethod=None  TranslationStandardOffset=0  TranslationLengthUnit=mm  TranslationStandardAxis=+Z  TranslationCartesianOffset=0  TranslationROffset=140  TranslationROffsetUnits=m  TranslationZOffset=0  TranslationZOffsetUnits=m  TranslationThetaOffset=0  TranslationThetaOffsetUnits=deg  RotationMethod=RotationMatrix  RotationAngleUnits=deg  RotationStandardAxis=+Z  RotationAngle=30  RotationArbitraryAxis=0  FollAlignAxisA=+X  BaseAlignAxisA=+Y  FollAlignAxisB=+Y  BaseAlignAxisB=+Z  RotationSequenceAxes=BaseAxes  RotationSequence=XYX  RotationSequenceAngles=[0 0 0]  RotationSequenceAnglesUnits=deg  RotationMatrix=stewart.lower_leg(3).rotation
  Transform Sphere_9 : sm_lib/Frames and Transforms/Rigid Transform  TranslationMethod=None  TranslationStandardOffset=0  TranslationLengthUnit=mm  TranslationStandardAxis=+Z  TranslationCartesianOffset=0  TranslationROffset=140  TranslationROffsetUnits=m  TranslationZOffset=0  TranslationZOffsetUnits=m  TranslationThetaOffset=0  TranslationThetaOffsetUnits=deg  RotationMethod=RotationMatrix  RotationAngleUnits=deg  RotationStandardAxis=+Z  RotationAngle=30  RotationArbitraryAxis=0  FollAlignAxisA=+X  BaseAlignAxisA=+Y  FollAlignAxisB=+Y  BaseAlignAxisB=+Z  RotationSequenceAxes=BaseAxes  RotationSequence=XYX  RotationSequenceAngles=[0 0 0]  RotationSequenceAnglesUnits=deg  RotationMatrix=stewart.lower_leg(4).rotation
  Bottom Leg_1 : PMIOPort  Side=Right
  Bottom Leg_2 : PMIOPort  Port=2  Side=Right
  Bottom Leg_3 : PMIOPort  Port=3  Side=Right
  Bottom Leg_4 : PMIOPort  Port=4  Side=Right
  Bottom Leg_5 : PMIOPort  Port=5  Side=Right
  Bottom Leg_6 : PMIOPort  Port=6  Side=Right
  World_Bottom : PMIOPort  Port=7  Side=Left
  connections:
  Transform Pos_base_2/LConn1 -- Transform Pos_base_3/LConn1 -- Transform Pos_base_4/LConn1 -- Transform Pos_base_6/LConn1 -- Transform Pos_base_5/LConn1 -- Bottom_Plate/LConn1 -- Transform Pos_base_1/LConn1
  Bottom Leg_1/RConn1 -- Transform Sphere_12/RConn1
  Transform Sphere_10/LConn1 -- Transform Sphere_5/RConn1
  Transform Sphere_9/LConn1 -- Transform Sphere_4/RConn1
  Transform Sphere_8/LConn1 -- Transform Sphere_3/RConn1
  Transform Sphere_7/RConn1 -- Bottom Leg_2/RConn1
  Transform Sphere_11/RConn1 -- Bottom Leg_6/RConn1
  Transform Sphere_6/LConn1 -- Sphere Bottom_6/LConn1
  Sphere Bottom_4/RConn1 -- Transform Pos_base_4/RConn1
  Transform Sphere_4/LConn1 -- Sphere Bottom_4/LConn1
  Sphere Bottom_1/RConn1 -- Transform Pos_base_1/RConn1
  Sphere Bottom_1/LConn1 -- Transform Sphere_1/LConn1
  Transform Sphere_9/RConn1 -- Bottom Leg_4/RConn1
  Sphere Bottom_5/RConn1 -- Transform Pos_base_5/RConn1
  Transform Sphere_10/RConn1 -- Bottom Leg_5/RConn1
  Transform Sphere_5/LConn1 -- Sphere Bottom_5/LConn1
  Sphere Bottom_3/RConn1 -- Transform Pos_base_3/RConn1
  Transform Sphere_3/LConn1 -- Sphere Bottom_3/LConn1
  Sphere Bottom_2/RConn1 -- Transform Pos_base_2/RConn1
  Transform Sphere_7/LConn1 -- Transform Sphere_2/RConn1
  Transform Sphere_2/LConn1 -- Sphere Bottom_2/LConn1
  Transform Sphere_12/LConn1 -- Transform Sphere_1/RConn1
  Transform Sphere_8/RConn1 -- Bottom Leg_3/RConn1
  Transform Sphere_11/LConn1 -- Transform Sphere_6/RConn1
  Sphere Bottom_6/RConn1 -- Transform Pos_base_6/RConn1
  Bottom_Plate/RConn1 -- World_Bottom/RConn1

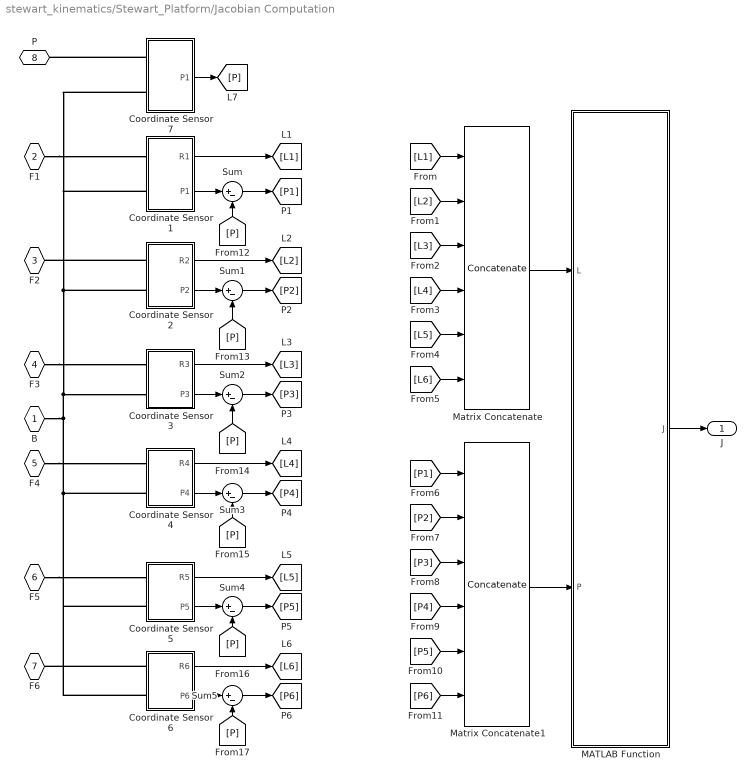
== system stewart_kinematics/Stewart_Platform/Jacobian Computation ==
  Coordinate Sensor 1 : Subsystem
  Coordinate Sensor 2 : Subsystem
  Coordinate Sensor 3 : Subsystem
  Coordinate Sensor 4 : Subsystem
  Coordinate Sensor 5 : Subsystem
  Coordinate Sensor 6 : Subsystem
  Coordinate Sensor 7 : Subsystem
  MATLAB Function : MATLAB Function  TreatAsAtomicUnit=on
  Matrix Concatenate : Concatenate  NumInputs=6  Mode=Multidimensional array  ConcatenateDimension=2
  Matrix Concatenate1 : Concatenate  NumInputs=6  Mode=Multidimensional array  ConcatenateDimension=2
  Sum{,1..5} (6 alike) : Sum  Inputs=|+-
  B : PMIOPort  Side=Left
  F1 : PMIOPort  Port=2  Side=Left
  F2 : PMIOPort  Port=3  Side=Left
  F3 : PMIOPort  Port=4  Side=Left
  F4 : PMIOPort  Port=5  Side=Left
  F5 : PMIOPort  Port=6  Side=Left
  F6 : PMIOPort  Port=7  Side=Left
  P : PMIOPort  Port=8  Side=Right
  J : Outport
  wires:
  [P] -> Sum5/2
  [P] -> Sum4/2
  [P] -> Sum3/2
  [P] -> Sum2/2
  [P] -> Sum1/2
  [P] -> Sum/2
  Coordinate Sensor 7/1(P1) -> [P]
  Coordinate Sensor 2/2(P2) -> Sum1/1
  Sum1/1 -> [P2]
  Coordinate Sensor 6/2(P6) -> Sum5/1
  Sum5/1 -> [P6]
  Coordinate Sensor 5/2(P5) -> Sum4/1
  Sum4/1 -> [P5]
  Coordinate Sensor 4/2(P4) -> Sum3/1
  Sum3/1 -> [P4]
  Coordinate Sensor 3/2(P3) -> Sum2/1
  Sum2/1 -> [P3]
  Sum/1 -> [P1]
  [P6] -> Matrix Concatenate1/6
  [P5] -> Matrix Concatenate1/5
  [P4] -> Matrix Concatenate1/4
  [P3] -> Matrix Concatenate1/3
  [P2] -> Matrix Concatenate1/2
  [P1] -> Matrix Concatenate1/1
  Coordinate Sensor 1/2(P1) -> Sum/1
  [L6] -> Matrix Concatenate/6
  [L4] -> Matrix Concatenate/4
  [L5] -> Matrix Concatenate/5
  [L3] -> Matrix Concatenate/3
  [L2] -> Matrix Concatenate/2
  [L1] -> Matrix Concatenate/1
  Coordinate Sensor 6/1(R6) -> [L6]
  Coordinate Sensor 5/1(R5) -> [L5]
  Coordinate Sensor 4/1(R4) -> [L4]
  Coordinate Sensor 3/1(R3) -> [L3]
  Coordinate Sensor 2/1(R2) -> [L2]
  Coordinate Sensor 1/1(R1) -> [L1]
  Matrix Concatenate1/1 -> MATLAB Function/2(P)
  MATLAB Function/1(J) -> J/1
  Matrix Concatenate/1 -> MATLAB Function/1(L)
  connections:
  Coordinate Sensor 7/LConn1 -- P/RConn1
  Coordinate Sensor 6/LConn1 -- F6/RConn1
  Coordinate Sensor 4/LConn2 -- Coordinate Sensor 6/LConn2 -- Coordinate Sensor 5/LConn2 -- Coordinate Sensor 3/LConn2 -- Coordinate Sensor 2/LConn2 -- Coordinate Sensor 1/LConn2 -- Coordinate Sensor 7/LConn2 -- B/RConn1
  Coordinate Sensor 2/LConn1 -- F2/RConn1
  F5/RConn1 -- Coordinate Sensor 5/LConn1
  F4/RConn1 -- Coordinate Sensor 4/LConn1
  F3/RConn1 -- Coordinate Sensor 3/LConn1
  F1/RConn1 -- Coordinate Sensor 1/LConn1
